simulink model "GUI_model"  (R2015a)
settings: Solver=ode23  StartTime=0.0  StopTime=10.0  RelTol=1e-3
libraries: nesl_utility x3, fl_lib x1
settings Model: Creator=DELL  LastModifiedBy=DELL
settings SolverCC: ZeroCrossControl=DisableAll

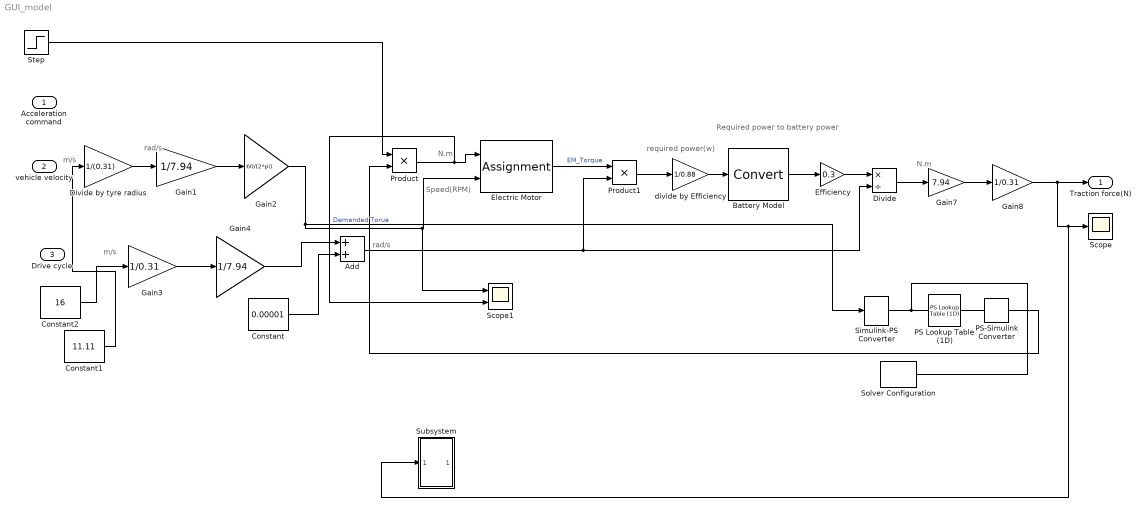
== system GUI_model ==
  note: m/s
  note: Required power to battery power
  note: m/s
  note: rad/s
  note: N.m
  note: required
      | power(w)
  note: N.m
  note: rad/s
  note: Speed(RPM)
  "Acceleration command " : Inport
  vehicle velocity : Inport  Port=2
  Drive cycle : Inport  Port=3
  Add : Sum
  Battery Model : DataTypeConversion
  Constant : Constant  Value=0.00001
  Constant1 : Constant  Value=11.11
  Constant2 : Constant  Value=16
  Divide : Product  Inputs=*/
  Divide by tyre radius : Gain  Gain=1/(0.31)
  Efficiency : Gain  Gain=0.3
  "Electric Motor " : Assignment  DiagnosticForDimensions=Warning
  Gain1 : Gain  Gain=1/7.94
  Gain2 : Gain  Gain=60/(2*pi)
  Gain3 : Gain  Gain=1/0.31
  Gain4 : Gain  Gain=1/7.94
  Gain7 : Gain  Gain=7.94
  Gain8 : Gain  Gain=1/0.31
  PS Lookup Table (1D) : fl_lib/Physical Signals/Lookup Tables/PS Lookup Table (1D)  x_t=[500, 1500]  y_t=[16.5, 5.5]  interp_method=1  extrap_method=1
  PS-Simulink Converter : nesl_utility/PS-Simulink Converter  PhysicalDomain=network_engine_domain  SubClassName=ps_output  LeftPortType=input  RightPortType=output  PseudoPeriodic=off  Frequencies=[]  Unit=1  AffineConversion=off
  Product : Product
  Product1 : Product
  Scope : Scope
  Scope1 : Scope  NumInputPorts=2
      settings: YMin=-5~-5  YMax=5~5
  Simulink-PS Converter : nesl_utility/Simulink-PS Converter  PhysicalDomain=network_engine_domain  SubClassName=ps_input  LeftPortType=input  RightPortType=output  PseudoPeriodic=off  Frequencies=[]  NoiseDistribution=none  NoiseParameters=[]  Unit=1  AffineConversion=off  InputFiltering=off  SimscapeFilterOrder=1  InputFilterTimeConstant=0.001  UdotUserProvided=1
  Solver Configuration : nesl_utility/Solver Configuration  PhysicalDomain=network_engine_domain  SubClassName=solver  LeftPortType=input  RightPortType=generic  Accelerate=off  Tones=[]  Harmonics=[]  SimulateNoise=off  Profile=off  UseLocalSampling=off  EnableSwitchedLinearOptims=on  FrequencyDomain=off  UseCCode=off  RelTol=0.001  AbsTol=1e-06  MinStep=1e-09  ToWorkspace=off  RevertToSquareIcSolve=off  NumHomotopyIterations=100  DoDC=off  ResidualTolerance=1e-09  UseLocalSolver=off  LocalSolverChoice=NE_BACKWARD_EULER_ADVANCER  LocalSolverSampleTime=0.001  DoFixedCost=off  MaxNonlinIter=3  MaxModeIter=2  LinearAlgebra=Sparse  DelaysMemoryBudget=1024  AutomaticFiltering=on  FilteringTimeConstant=0.001
  Step : Step  Time=5  Before=1  After=-2  SampleTime=0
  Subsystem : Subsystem
  divide by Efficiency : Gain  Gain=1/0.88
  Traction force(N) : Outport
  wires:
  Divide by tyre radius/1 -> Gain1/1
  Gain1/1 -> Gain2/1
  PS-Simulink Converter/1 -> Product/2
  Step/1 -> Product/1
  "Electric Motor "/1 -> Product1/1  "EM_Torque"
  Constant2/1 -> Gain3/1
  Gain3/1 -> Gain4/1
  Gain4/1 -> Add/1
  Constant/1 -> Add/2
  Product1/1 -> divide by Efficiency/1
  divide by Efficiency/1 -> Battery Model/1
  Battery Model/1 -> Efficiency/1
  Efficiency/1 -> Divide/1
  Add/1 -> Divide/2, Product1/2
  Divide/1 -> Gain7/1
  Gain7/1 -> Gain8/1
  Gain8/1 -> Subsystem/1(In1), Scope/1, Traction force(N)/1
  Product/1 -> Scope1/2, "Electric Motor "/1  "Demanded Torue"
  Gain2/1 -> Simulink-PS Converter/1, Scope1/1, "Electric Motor "/2
  Constant1/1 -> Divide by tyre radius/1
  connections:
  Simulink-PS Converter/RConn1 -- Solver Configuration/RConn1 -- PS Lookup Table (1D)/LConn1
  PS Lookup Table (1D)/RConn1 -- PS-Simulink Converter/LConn1

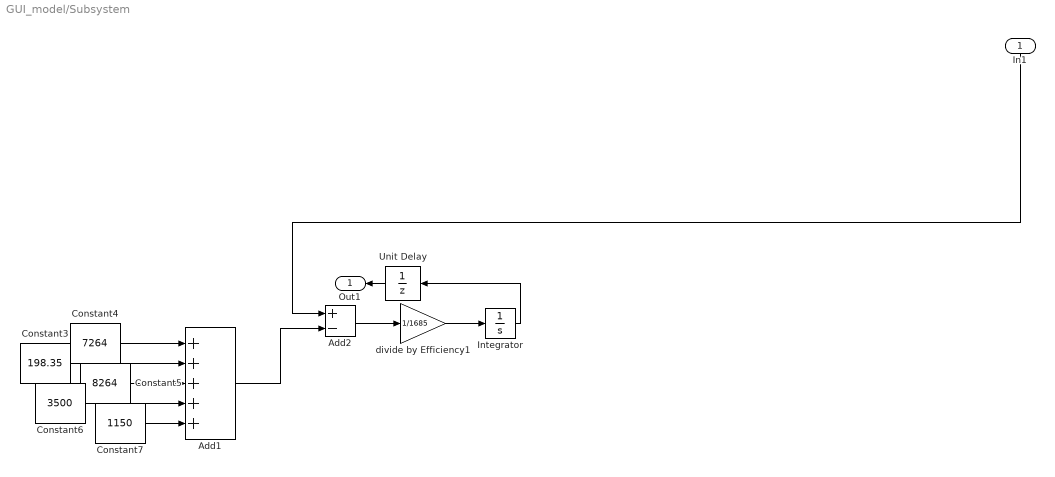
== system GUI_model/Subsystem ==
  In1 : Inport
  Add1 : Sum  Inputs=+++++
  Add2 : Sum  Inputs=+-
  Constant3 : Constant  Value=198.35
  Constant4 : Constant  Value=7264
  Constant5 : Constant  Value=8264
  Constant6 : Constant  Value=3500
  Constant7 : Constant  Value=1150
  Integrator : Integrator
  Unit Delay : UnitDelay  InitialCondition=11
  divide by Efficiency1 : Gain  Gain=1/1685
  Out1 : Outport
  wires:
  divide by Efficiency1/1 -> Integrator/1
  Constant3/1 -> Add1/2
  Integrator/1 -> Unit Delay/1
  Unit Delay/1 -> Out1/1
  In1/1 -> Add2/1
  Constant5/1 -> Add1/3
  Constant4/1 -> Add1/1
  Add2/1 -> divide by Efficiency1/1
  Constant6/1 -> Add1/4
  Constant7/1 -> Add1/5
  Add1/1 -> Add2/2
